simulink model "TricopterModel"  (R2014b)
settings: Solver=ode3  StartTime=0.0  StopTime=10  FixedStep=T_sim  MaxStep=0.01  RelTol=1e-5
values from neighbouring files (symbols this model uses):
  A_x = 0.015    [SetupComplete.m]
  A_y = A_x    (= 0.015)    [SetupComplete.m]
  A_z = 0.16    [SetupComplete.m]
  C_x = 1.2    [SetupComplete.m]
  C_y = C_x    (= 1.2)    [SetupComplete.m]
  C_z = 2.2    [SetupComplete.m]
  CG_0 = [0,0,0.02]'    [SetupComplete.m]
  eta_23 = deg2rad(-1.42)    [Run3Copter.m]
  h = 0.08    [SetupComplete.m]
  h_M = 0.064    [SetupComplete.m]
  I_BAC_0 = [ Ix,0,Ixz;0,Iy,0;Ixz,0,Iz]    [SetupComplete.m]
  Initial_Omegas = Omega_hover    [Run3Copter.m]
  Initial_Torques = Torque_hover    [Run3Copter.m]
  l = 0.345    [SetupComplete.m]
  l_arm = 0.264    [SetupComplete.m]
  m = 3.51    [SetupComplete.m]
  m_0 = 2.61    [SetupComplete.m]
  m_M = 0.300    (= 0.3)    [SetupComplete.m]
  rho = 1.15    [SetupComplete.m]
  Rotation_sign = [ 1,-1,-1]    [SetupComplete.m]
  Throttle_Hover = 0.745    [Run3Copter.m]
undefined symbols (not defined in the file or in its folder): DOWN_0, EAST_0, NORTH_0, P_0, Q_0, R_0, U_0, V_0, W_0
libraries: simulink_extras x7, XXCopter x4, XXCopter_C x3, aerolibutil x2, aerolib6dofsys x1
(part 2 of 2)

== matlab function TricopterModel/3 Copter Complete/6dof Eqs of motion/SVFI_to_SVFb ==
  data: X_e input; V_e input; X_e_out output; V_b output; omega_b output; Euler_Ang input; Euler_Ang_Dot input; q output
function [X_e_out,V_b, omega_b ,q]=SVFI_to_SVFb(X_e,V_e, Euler_Ang,Euler_Ang_Dot)

xp=V_e(1);
yp=V_e(2);
zp=V_e(3);

phi=Euler_Ang(1);
theta=Euler_Ang(2);
psi=Euler_Ang(3);
phip=Euler_Ang_Dot(1);
thetap=Euler_Ang_Dot(2);
psip=Euler_Ang_Dot(3);

%%
X_e_out=X_e;

q = QuaternionfromEuler(phi,theta,psi); 



HamOut=HamiltonProduct([q(1);-q(2);-q(3);-q(4)],HamiltonProduct([0;xp;yp;zp],[q(1);q(2);q(3);q(4)]) );% q* . v . q
V_b=HamOut(2:4);

omega_b=[phip-psip*sin(theta)  ;
         thetap*cos(phi)+psip*cos(theta)*sin(phi);
            -thetap*sin(phi)+psip*cos(theta)*cos(phi)  ];% Ya que es solo una operacion aislada utilizaremos la ecuaciones con rel trigonometricas
end
function [q]=QuaternionfromEuler(phi,theta,psi)
% options=optimset('MaxFunEvals',3000);
% q=fsolve(@QUATERNIONEULER,[0.6,0.4,0.5,0.4]); % Hay que acertar con los angulos poniendo diferentes valores iniciales del quaternion
%     function F=QUATERNIONEULER(q)
%         F=[ tan(phi)-(2*q(3)*q(4)-2*q(1)*q(2))/(2*q(1)^2+2*q(4)^2-1)  ;
%             sin(-theta)-2*q(2)*q(4)-2*q(1)*q(3);
%             tan(psi)-(2*q(2)*q(3)-2*q(1)*q(4))/(2*q(1)^2+2*q(2)^2-1);
%             q(1)^2+q(2)^2+q(3)^2+q(4)^2-1];
%     end  % Este algoritmo da q* !!!!!

q=[ cos(psi/2)*cos(theta/2)*cos(phi/2)+ sin(psi/2)*sin(theta/2)*sin(phi/2) ;
      cos(psi/2)*cos(theta/2)*sin(phi/2)- sin(psi/2)*sin(theta/2)*cos(phi/2) ;
       cos(psi/2)*sin(theta/2)*cos(phi/2)+ sin(psi/2)*cos(theta/2)*sin(phi/2)   ;
        sin(psi/2)*cos(theta/2)*cos(phi/2)- cos(psi/2)*sin(theta/2)*sin(phi/2)      ]; % Esto nos da q !!!
end

== matlab function TricopterModel/3 Copter Complete/6dof Eqs of motion/SV_F_b_to_SV_FI ==
  data: V_b input; q_dot input; q input; V_e output; euler output; euler_dot output
function [V_e,euler,euler_dot]   = SV_F_b_to_SV_FI(  V_b, q_dot,q)

xp=V_b(1);
yp=V_b(2);
zp=V_b(3);

%% Velocity and position in Earth Frame   q . v . q*

SolProd=HamiltonProduct([q(1);q(2);q(3);q(4)],HamiltonProduct([0;xp;yp;zp],[q(1);-q(2);-q(3);-q(4)]) );
V_e=SolProd(2:4);

%% Actitud en Angulos de Euler y sus derivadas. 
euler=[0,0,0]';
euler(1) = atan2(2*q(3)*q(4)+2*q(1)*q(2),2*q(1)^2+2*q(4)^2-1 ); % phi
euler(2) = -asin( 2*q(2)*q(4)-2*q(1)*q(3) ); %  theta
euler(3) = atan2( 2*q(2)*q(3)+2*q(1)*q(4),2*q(1)^2+2*q(2)^2-1 ); %  psi

euler_dot=[0,0,0]';
euler_dot(1,1) = 2/(1+( (2*q(3)*q(4)+2*q(1)*q(2))/(2*q(1)^2+2*q(4)^2-1)  )^2)*[ -(2*q(1)^2*q(2)+ 4*q(1)*q(3)*q(4)-2*q(2)*q(4)^2+q(2))  ,  q(1)*(2*q(1)^2+2*q(4)^2-1)  ,  q(4)*(2*q(1)^2+2*q(4)^2-1)  ,  -(-2*q(1)^2*q(3) +4*q(1)*q(2)*q(4)+2*q(3)*q(4)^2+q(3) ) ]*q_dot.* 1/(2*q(1)^2+2*q(4)^2-1)^2; % Derivada de phi
euler_dot(2,1) = -2/( sqrt(1-4*(q(2)*q(4)-q(1)*q(3))^2)  )*[-q(3),q(4),-q(1),q(2)]*q_dot;  % Theta prima
euler_dot(3,1) = 2/(1+( (2*q(2)*q(3)+2*q(1)*q(4))/(2*q(1)^2+2*q(2)^2-1)  )^2)*[  -(2*q(1)^2*q(4)+4*q(1)*q(2)*q(3)-2*q(2)^2*q(4)+q(4)  ) , 1/2*(q(3)*(4*q(1)^2-4*q(2)^2-2)-8*q(1)*q(2)*q(4) )  ,  q(2)*(2*q(1)^2+2*q(2)^2-1)  , q(1)*(2*q(1)^2+2*q(2)^2-1) ]*q_dot.*1/(2*q(1)^2+2*q(2)^2-1)^2;  % Psi prima



end

== matlab function TricopterModel/3 Copter Complete/Mass Properties/Arm Inertia ==
  data: T1_FAFb input; T2_FAFb input; T3_FAFb input; I_M output; l parameter; h_M parameter; m_M parameter; r1_M output; r2_M output; r3_M output
function [I_M,r1_M,r2_M,r3_M]  = Arm1_inertia(T1_FAFb,T2_FAFb,T3_FAFb, l, h_M, m_M)


r1_M=[l;0;0]+T1_FAFb*[0;0;-h_M];
r2_M=[-1/2*l;sqrt(3)/2*l;0]+T2_FAFb*[0;0;-h_M];
r3_M=[-1/2*l;-sqrt(3)/2*l;0]+T3_FAFb*[0;0;-h_M];


I_M1 = m_M*[ r1_M(2)^2+r1_M(3)^2,r1_M(1)*r1_M(2),r1_M(1)*r1_M(3);...
            r1_M(1)*r1_M(2), r1_M(1)^2+r1_M(3)^2, r1_M(2)*r1_M(3);...
            r1_M(1)*r1_M(3),r1_M(2)*r1_M(3), r1_M(1)^2+r1_M(2)^2];
I_M2 = m_M*[ r2_M(2)^2+r2_M(3)^2,r2_M(1)*r2_M(2),r2_M(1)*r2_M(3);...
            r2_M(1)*r2_M(2), r2_M(1)^2+r2_M(3)^2, r2_M(2)*r2_M(3);...
            r2_M(1)*r2_M(3),r2_M(2)*r2_M(3), r2_M(1)^2+r2_M(2)^2];
I_M3 = m_M*[ r3_M(2)^2+r3_M(3)^2,r3_M(1)*r3_M(2),r3_M(1)*r3_M(3);...
            r3_M(1)*r3_M(2), r3_M(1)^2+r3_M(3)^2, r3_M(2)*r3_M(3);...
            r3_M(1)*r3_M(3),r3_M(2)*r3_M(3), r3_M(1)^2+r3_M(2)^2];

I_M = I_M1+I_M2+I_M3;

== matlab function TricopterModel/Atomic Subsystem/3Copter_4_NDI/6dof Eqs of motion/Position Eqs ==
  data: A_b output size=[3,1]; Vb input size=[3,1]; omega_b input size=[3,1]; omega_b_dot input size=[3,1]; Forces input size=[3,1]; m input size=1; CG input size=[3,1]
function A_b  = PositionEqs(Vb,omega_b,omega_b_dot, Forces,m, CG)



 
A_b =  1/m*( Forces ) - cross(omega_b,Vb) - cross(omega_b, cross(omega_b,CG)) -cross(omega_b_dot,CG)  ;

== matlab function TricopterModel/Atomic Subsystem/3Copter_4_NDI/6dof Eqs of motion/Rotational eqs ==
  data: omega_dot output; omega_b input; Moments input; I_BAC input
function omega_dot  = Rotational_Eq(omega_b,Moments, I_BAC)



omega_dot =  I_BAC\( Moments - cross(omega_b,I_BAC*omega_b)  );

== matlab function TricopterModel/Atomic Subsystem/3Copter_4_NDI/6dof Eqs of motion/SV_F_b_to_SV_FI ==
  data: q input; V_b input; V_e output
function V_e= SV_F_b_to_SV_FI(  q,V_b)

xp=V_b(1);
yp=V_b(2);
zp=V_b(3);

%% Velocity and position in Earth Frame   q . v . q*

SolProd=HamiltonProduct([q(1);q(2);q(3);q(4)],HamiltonProduct([0;xp;yp;zp],[q(1);-q(2);-q(3);-q(4)]) );
V_e=SolProd(2:4);


end

== matlab function TricopterModel/Atomic Subsystem/3Copter_4_NDI/6dof Eqs of motion/q_dot/Quaternion_dot ==
  data: omega_b input; q_dot output; q input
function q_dot = Quaternion_dot(omega_b,q)


q_dot = 1/2*HamiltonProduct(q,[0;omega_b]);

== matlab function TricopterModel/Atomic Subsystem/3Copter_4_NDI/Aerodynamics body Force and Moment1 ==
  data: V_b input; F_a_b output; M_a_b output; rho parameter; C_x parameter; C_y parameter; C_z parameter; A_x parameter; A_y parameter; A_z parameter
function [F_a_b,M_a_b]   = Aero_body_Forces_and_Mom( V_b, rho,C_x,C_y,C_z,A_x,A_y,A_z)


F_a_b=1/2.0*rho*(V_b*V_b')*[C_x*A_x;C_y*A_y;C_z*A_z].*( - V_b./(norm(V_b)+eps) );
M_a_b=[0;0;0];
end

== matlab function TricopterModel/Atomic Subsystem/3Copter_4_NDI/Gravity Force and Moment ==
  data: q input size=[4,1]; F_g_b output; M_g_b output; mass input; CG input; g parameter
function [F_g_b,M_g_b]   = Grav_Forces_and_Mom( q,mass,CG, g)

Prod=HamiltonProduct([q(1);-q(2);-q(3);-q(4)],HamiltonProduct([0;0;0;mass*g],[q(1);q(2);q(3);q(4)]) ); % q* . g .q

F_g_b= Prod(2:4);
M_g_b=cross(CG,F_g_b);
end

== matlab function TricopterModel/Atomic Subsystem/3Copter_4_NDI/Mass Properties/Arm Inertia ==
  data: T1_FAFb input; T2_FAFb input; T3_FAFb input; I_M output; l parameter; h_M parameter; m_M parameter; r1_M output; r2_M output; r3_M output
function [I_M,r1_M,r2_M,r3_M]  = Arm1_inertia(T1_FAFb,T2_FAFb,T3_FAFb, l, h_M, m_M)


r1_M=[l;0;0]+T1_FAFb*[0;0;-h_M];
r2_M=[-1/2*l;sqrt(3)/2*l;0]+T2_FAFb*[0;0;-h_M];
r3_M=[-1/2*l;-sqrt(3)/2*l;0]+T3_FAFb*[0;0;-h_M];


I_M1 = m_M*[ r1_M(2)^2+r1_M(3)^2,r1_M(1)*r1_M(2),r1_M(1)*r1_M(3);...
            r1_M(1)*r1_M(2), r1_M(1)^2+r1_M(3)^2, r1_M(2)*r1_M(3);...
            r1_M(1)*r1_M(3),r1_M(2)*r1_M(3), r1_M(1)^2+r1_M(2)^2];
I_M2 = m_M*[ r2_M(2)^2+r2_M(3)^2,r2_M(1)*r2_M(2),r2_M(1)*r2_M(3);...
            r2_M(1)*r2_M(2), r2_M(1)^2+r2_M(3)^2, r2_M(2)*r2_M(3);...
            r2_M(1)*r2_M(3),r2_M(2)*r2_M(3), r2_M(1)^2+r2_M(2)^2];
I_M3 = m_M*[ r3_M(2)^2+r3_M(3)^2,r3_M(1)*r3_M(2),r3_M(1)*r3_M(3);...
            r3_M(1)*r3_M(2), r3_M(1)^2+r3_M(3)^2, r3_M(2)*r3_M(3);...
            r3_M(1)*r3_M(3),r3_M(2)*r3_M(3), r3_M(1)^2+r3_M(2)^2];

I_M = I_M1+I_M2+I_M3;
